simulink model "sampleModel242"  (R2021b)
settings: Solver=VariableStepAuto  StartTime=0.0  StopTime=10.0  RelTol=1e-3
undefined symbols (not defined in the file or in its folder): DiscIntNeverNeededParam
libraries: simulink x20, slpidlib x4
settings Model: Creator=user  LastModifiedBy=user

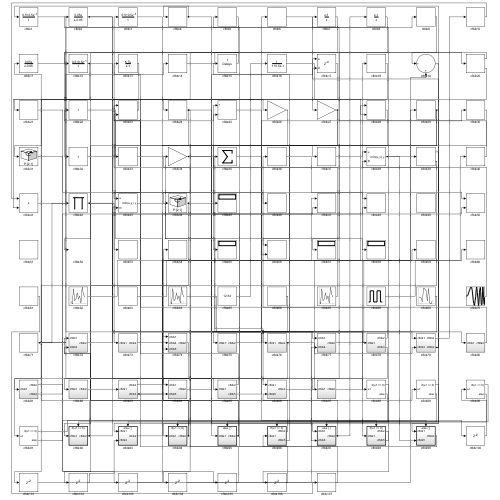
[thumbnail: Simulink's stored preview of the top-level diagram]
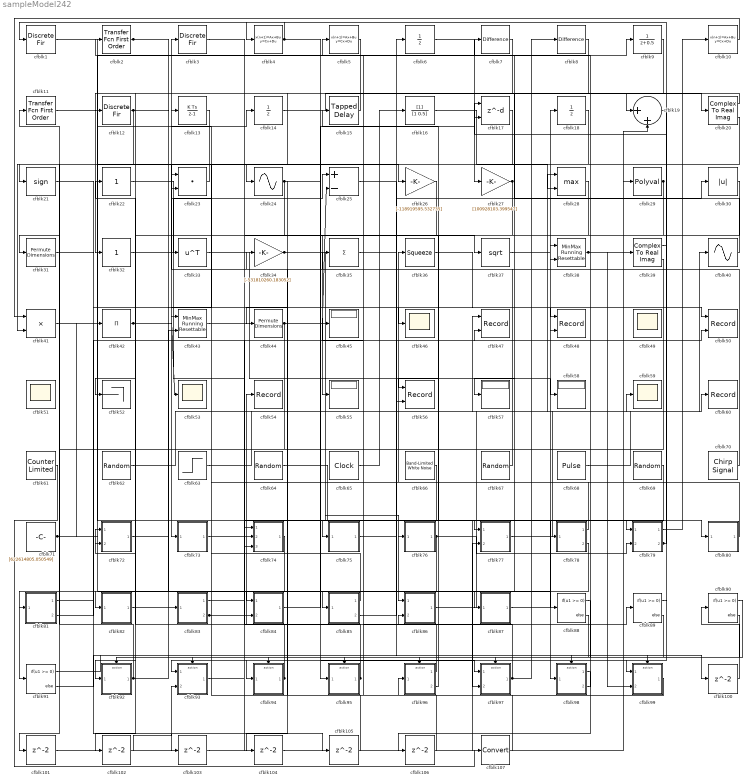
== system sampleModel242 ==
  cfblk1 : DiscreteFir  SampleTime=1
  cfblk10 : DiscreteStateSpace
  cfblk{100..106} (7 alike) : Delay  SampleTime=1
  cfblk107 : DataTypeConversion
  cfblk11 : simulink/Discrete/Transfer Fcn First Order  PoleZ=0.95  ICPrevOutput=0.0  DoSatur=off
  cfblk12 : DiscreteFir  SampleTime=1
  cfblk13 : DiscreteIntegrator  ICPrevOutput=DiscIntNeverNeededParam  ICPrevScaledInput=DiscIntNeverNeededParam
  cfblk14 : UnitDelay  HasFrameUpgradeWarning=on
  cfblk15 : simulink/Discrete/Tapped Delay  vinit=0.0  samptime=-1  NumDelays=1  DelayOrder=Oldest  includeCurrent=off
  cfblk16 : DiscreteFilter  SampleTime=1
  cfblk17 : Delay  DelayLengthSource=Input port  SampleTime=1
      settings: InputPortMap=u0,p1
  cfblk18 : UnitDelay  HasFrameUpgradeWarning=on
  cfblk19 : Sum  Inputs=|++
  cfblk2 : simulink/Discrete/Transfer Fcn First Order  PoleZ=0.95  ICPrevOutput=0.0  DoSatur=off
  cfblk20 : ComplexToRealImag
  cfblk21 : Signum
  cfblk22 : simulink/Math Operations/Slider Gain  gain=1  low=0  high=2
  cfblk23 : DotProduct  InputSameDT=on  OutDataTypeStr=Inherit: Inherit via internal rule
  cfblk24 : Sin  TimeSource=Use external signal  SampleTime=0
  cfblk25 : Sum  Inputs=+-
  cfblk26 : Gain  Gain=[-118919595.532735]
  cfblk27 : Gain  Gain=[100928103.399547]
  cfblk28 : MinMax  Function=max  Inputs=2
  cfblk29 : Polyval  Coefs=[ +2.081618890e-019, -1.441693666e-014, +4.719686976e-010, -8.536869453e-006, +1.621573104e-001, -8.087801117e+001 ]
  cfblk3 : DiscreteFir  SampleTime=1
  cfblk30 : Abs
  cfblk31 : PermuteDimensions
  cfblk32 : simulink/Math Operations/Slider Gain  gain=1  low=0  high=2
  cfblk33 : Math  Operator=transpose  SaturateOnIntegerOverflow=on
  cfblk34 : Gain  Gain=[-531810260.183052]
  cfblk35 : Sum  Inputs=+
  cfblk36 : Squeeze
  cfblk37 : Sqrt  SaturateOnIntegerOverflow=on
  cfblk38 : simulink/Math Operations/MinMax Running Resettable  Function=min  vinit=0.0
  cfblk39 : ComplexToRealImag
  cfblk4 : DiscreteStateSpace
  cfblk40 : Sin  TimeSource=Use external signal  SampleTime=0
  cfblk41 : Product  Inputs=**
  cfblk42 : Product  Inputs=*
  cfblk43 : simulink/Math Operations/MinMax Running Resettable  Function=min  vinit=0.0
  cfblk44 : PermuteDimensions
  cfblk{45,55,57..58} (4 alike) : Display
  cfblk{46,49,51,53,59} (5 alike) : Scope
      cfblk49 settings: Floating=on
      cfblk51 settings: Floating=on
  cfblk47 : Record  FileSettingsInternal="{\"entries\":[{\"content\":{\"excelSettings\":{\"content\":{},\"type\":\"Streamout.ExcelSettings\"}},\"type\":\"Streamout.FileSettingStorage\",\"uuid\":\"8466640d-3540-4ce9-993a-5f65f49446ff\"}],\"packageUris\":[\"http://schema.mathworks.com/mf0/streamout_blocks/R2020a\"],\"version\":\"1.0\"}"  Layout=[1 1]  SignalsInternal="{\"entries\":[{\"content\":{\"signals\":[{\"content\":{\"blockPath\":[\"sampleModel242/cfblk47\"],\"channel\":[],\"dimensions\":[1],\"domain\":\"sampleModel242/cfblk47\",\"lineColor\":\"#a2142f\",\"plots\":[1],\"port\":1,\"sid\":[\"\"],\"signalID\":9661,\"signalName\":\"cfblk63\"},\"type\":\"RecordBlkView.Signal\",\"uuid\":\"67ad4537-a0c7-4a78-aa5b-3ca15c563dde\"},{\"content\":{\"blockPath\":[\"sampleModel242/cfblk47\"],\"channel\":[],\"dimensions\":[1,1],\"domain\":\"sampleModel242/cfblk47\",\"lineColor\":\"#139fff\",\"plots\":[1],\"port\":2,\"sid\":[\"\"],\"signalID\":9665,\"signalName\":\"cfblk92\"},\"type\":\"RecordBlkView.Signal\",\"uuid\":\"e8972b09-f2da-4a53-9017-1d3f0a4a10ed\"}]},\"type\":\"RecordBlkView.InputSignals\",\"uuid\":\"aacada88-77af-4606-b280-0a5f38fbb807\"}],\"packageUris\":[\"http://schema.mathworks.com/mf0/streamout_blocks/R2020a\"],\"version\":\"1.0\"}"  VisualizationBindings="{\"xyplotplugin\":{\"info\":[{\"series\":[{\"bindingParametersList\":[{\"parameter\":\"X-Axis\",\"signalID\":9661,\"signalName\":\"cfblk63\"},{\"parameter\":\"Y-Axis\",\"signalID\":9665,\"signalName\":\"cfblk92\"}],\"seriesID\":40376}],\"subplotID\":1}]}}"  CompatibilityTag=XY
  cfblk48 : Record  FileSettingsInternal="{\"entries\":[{\"content\":{\"excelSettings\":{\"content\":{},\"type\":\"Streamout.ExcelSettings\"}},\"type\":\"Streamout.FileSettingStorage\",\"uuid\":\"c13b47bf-a8bf-41b9-80a1-0a6b1b0ceada\"}],\"packageUris\":[\"http://schema.mathworks.com/mf0/streamout_blocks/R2020a\"],\"version\":\"1.0\"}"  Layout=[1 1]  SignalsInternal="{\"entries\":[{\"content\":{\"signals\":[{\"content\":{\"blockPath\":[\"sampleModel242/cfblk48\"],\"channel\":[],\"dimensions\":[1,1],\"domain\":\"sampleModel242/cfblk48\",\"lineColor\":\"#a2142f\",\"plots\":[1],\"port\":1,\"sid\":[\"\"],\"signalID\":9669,\"signalName\":\"cfblk31\"},\"type\":\"RecordBlkView.Signal\",\"uuid\":\"329d8449-1276-47a0-bcc8-603c41fd3026\"},{\"content\":{\"blockPath\":[\"sampleModel242/cfblk48\"],\"channel\":[],\"dimensions\":[1],\"domain\":\"sampleModel242/cfblk48\",\"lineColor\":\"#139fff\",\"plots\":[1],\"port\":2,\"sid\":[\"\"],\"signalID\":9673,\"signalName\":\"cfblk83:2\"},\"type\":\"RecordBlkView.Signal\",\"uuid\":\"b307b965-bfc8-4c75-a60e-a0313d9c2b02\"}]},\"type\":\"RecordBlkView.InputSignals\",\"uuid\":\"3cab57f9-6900-416a-b86f-56591b424206\"}],\"packageUris\":[\"http://schema.mathworks.com/mf0/streamout_blocks/R2020a\"],\"version\":\"1.0\"}"  VisualizationBindings="{\"xyplotplugin\":{\"info\":[{\"series\":[{\"bindingParametersList\":[{\"parameter\":\"X-Axis\",\"signalID\":9669,\"signalName\":\"cfblk31\"},{\"parameter\":\"Y-Axis\",\"signalID\":9673,\"signalName\":\"cfblk83:2\"}],\"seriesID\":38915}],\"subplotID\":1}]}}"  CompatibilityTag=XY
  cfblk5 : DiscreteStateSpace
  cfblk50 : Record  FileSettingsInternal="{\"entries\":[{\"content\":{\"excelSettings\":{\"content\":{},\"type\":\"Streamout.ExcelSettings\"}},\"type\":\"Streamout.FileSettingStorage\",\"uuid\":\"6b25f1e0-3625-4cd8-9b2f-529eb5e0b0c7\"}],\"packageUris\":[\"http://schema.mathworks.com/mf0/streamout_blocks/R2020a\"],\"version\":\"1.0\"}"  Layout=[1 1]  SignalsInternal="{\"entries\":[{\"content\":{\"signals\":[{\"content\":{\"blockPath\":[\"sampleModel242/cfblk50\"],\"channel\":[],\"dimensions\":[1],\"domain\":\"sampleModel242/cfblk50\",\"lineColor\":\"#a2142f\",\"plots\":[1],\"port\":1,\"sid\":[\"\"],\"signalID\":9677,\"signalName\":\"cfblk36\"},\"type\":\"RecordBlkView.Signal\",\"uuid\":\"2faef9c5-9386-467e-8d00-879811eaf1a7\"},{\"content\":{\"blockPath\":[\"sampleModel242/cfblk50\"],\"channel\":[],\"dimensions\":[1],\"domain\":\"sampleModel242/cfblk50\",\"lineColor\":\"#139fff\",\"plots\":[1],\"port\":2,\"sid\":[\"\"],\"signalID\":9681,\"signalName\":\"cfblk81:2\"},\"type\":\"RecordBlkView.Signal\",\"uuid\":\"3fd7d5d3-1578-4a63-9d5f-ee0901e409a9\"}]},\"type\":\"RecordBlkView.InputSignals\",\"uuid\":\"3d327c85-3593-4bfd-8775-d910ec92d710\"}],\"packageUris\":[\"http://schema.mathworks.com/mf0/streamout_blocks/R2020a\"],\"version\":\"1.0\"}"  VisualizationBindings="{\"xyplotplugin\":{\"info\":[{\"series\":[{\"bindingParametersList\":[{\"parameter\":\"X-Axis\",\"signalID\":9677,\"signalName\":\"cfblk36\"},{\"parameter\":\"Y-Axis\",\"signalID\":9681,\"signalName\":\"cfblk81:2\"}],\"seriesID\":706}],\"subplotID\":1}]}}"  CompatibilityTag=XY
  cfblk52 : Terminator
  cfblk54 : Record  FileSettingsInternal="{\"entries\":[{\"content\":{\"excelSettings\":{\"content\":{},\"type\":\"Streamout.ExcelSettings\"}},\"type\":\"Streamout.FileSettingStorage\",\"uuid\":\"06190793-f5fc-415c-b838-8303df1b911b\"}],\"packageUris\":[\"http://schema.mathworks.com/mf0/streamout_blocks/R2020a\"],\"version\":\"1.0\"}"  SignalsInternal="{\"entries\":[{\"content\":{\"signals\":[{\"content\":{\"blockPath\":[\"sampleModel242/cfblk54\"],\"channel\":[],\"dimensions\":[1],\"domain\":\"sampleModel242/cfblk54\",\"lineColor\":\"#ff13a6\",\"plots\":[1],\"port\":1,\"sid\":[\"\"],\"signalID\":9685,\"signalName\":\"cfblk94\"},\"type\":\"RecordBlkView.Signal\",\"uuid\":\"6a6a1d66-a567-4c36-91e1-80c7a0c5bc7a\"}]},\"type\":\"RecordBlkView.InputSignals\",\"uuid\":\"c8db5507-b214-4169-ac9a-3b7f1f8d503c\"}],\"packageUris\":[\"http://schema.mathworks.com/mf0/streamout_blocks/R2020a\"],\"version\":\"1.0\"}"  VisualizationBindings="{\"sparklinesplugin\":{\"info\":[{\"bindingParametersList\":[],\"subplotID\":1}]}}"
  cfblk56 : Record  FileSettingsInternal="{\"entries\":[{\"content\":{\"excelSettings\":{\"content\":{},\"type\":\"Streamout.ExcelSettings\"}},\"type\":\"Streamout.FileSettingStorage\",\"uuid\":\"80c68350-c5d5-4745-a822-7bd470e9d639\"}],\"packageUris\":[\"http://schema.mathworks.com/mf0/streamout_blocks/R2020a\"],\"version\":\"1.0\"}"  Layout=[1 1]  SignalsInternal="{\"entries\":[{\"content\":{\"signals\":[{\"content\":{\"blockPath\":[\"sampleModel242/cfblk56\"],\"channel\":[],\"dimensions\":[1],\"domain\":\"sampleModel242/cfblk56\",\"lineColor\":\"#a2142f\",\"plots\":[1],\"port\":1,\"sid\":[\"\"],\"signalID\":9689,\"signalName\":\"cfblk29\"},\"type\":\"RecordBlkView.Signal\",\"uuid\":\"3f9a410f-4a9b-4b88-868e-e92ce524b347\"},{\"content\":{\"blockPath\":[\"sampleModel242/cfblk56\"],\"channel\":[],\"dimensions\":[1],\"domain\":\"sampleModel242/cfblk56\",\"lineColor\":\"#139fff\",\"plots\":[1],\"port\":2,\"sid\":[\"\"],\"signalID\":9693,\"signalName\":\"cfblk35\"},\"type\":\"RecordBlkView.Signal\",\"uuid\":\"47182436-db97-462b-940f-56f22781204b\"}]},\"type\":\"RecordBlkView.InputSignals\",\"uuid\":\"28bf4cd6-305f-4118-8603-ea67f9f3f1eb\"}],\"packageUris\":[\"http://schema.mathworks.com/mf0/streamout_blocks/R2020a\"],\"version\":\"1.0\"}"  VisualizationBindings="{\"xyplotplugin\":{\"info\":[{\"series\":[{\"bindingParametersList\":[{\"parameter\":\"X-Axis\",\"signalID\":9689,\"signalName\":\"cfblk29\"},{\"parameter\":\"Y-Axis\",\"signalID\":9693,\"signalName\":\"cfblk35\"}],\"seriesID\":40562}],\"subplotID\":1}]}}"  CompatibilityTag=XY
  cfblk6 : UnitDelay  HasFrameUpgradeWarning=on
  cfblk60 : Record  FileSettingsInternal="{\"entries\":[{\"content\":{\"excelSettings\":{\"content\":{},\"type\":\"Streamout.ExcelSettings\"}},\"type\":\"Streamout.FileSettingStorage\",\"uuid\":\"ac3e01c3-e921-4d05-880d-693c9b2be958\"}],\"packageUris\":[\"http://schema.mathworks.com/mf0/streamout_blocks/R2020a\"],\"version\":\"1.0\"}"  SignalsInternal="{\"entries\":[{\"content\":{\"signals\":[{\"content\":{\"blockPath\":[\"sampleModel242/cfblk60\"],\"channel\":[],\"dimensions\":[1],\"domain\":\"sampleModel242/cfblk60\",\"lineColor\":\"#77ac30\",\"plots\":[1],\"port\":1,\"sid\":[\"\"],\"signalID\":9657,\"signalName\":\"cfblk73\"},\"type\":\"RecordBlkView.Signal\",\"uuid\":\"ee10d19c-2b42-44d8-8030-24d641aff3a6\"}]},\"type\":\"RecordBlkView.InputSignals\",\"uuid\":\"6dbc1fc7-41f6-4a64-bb1e-672c8c773d34\"}],\"packageUris\":[\"http://schema.mathworks.com/mf0/streamout_blocks/R2020a\"],\"version\":\"1.0\"}"  VisualizationBindings="{\"sparklinesplugin\":{\"info\":[{\"bindingParametersList\":[],\"subplotID\":1}]}}"
  cfblk61 : simulink/Sources/Counter Limited  uplimit=[647.000000]  tsamp=-1
  cfblk62 : UniformRandomNumber  Minimum=[-3232928567.587387]  Maximum=[4444264149.465066]  Seed=[1192027.000000]  SampleTime=0.1
  cfblk63 : Step  Time=[34.000000]  Before=[160858895.694501]  After=[813002846.290973]  SampleTime=0
  cfblk64 : UniformRandomNumber  Minimum=[-4185575344.574016]  Maximum=[9583603799.572458]  Seed=[1929106.000000]  SampleTime=0.1
  cfblk65 : DigitalClock
  cfblk66 : simulink/Sources/Band-Limited White Noise  Cov=[5099447589.018917]  Ts=0.1  seed=[2237415079.000000]
  cfblk67 : UniformRandomNumber  Minimum=[-6418738320.620914]  Maximum=[7113492972.441939]  Seed=[24566985.000000]  SampleTime=0.1
  cfblk68 : DiscretePulseGenerator  PulseType=Time based  Amplitude=[-591785427.766708]  Period=[98460536.017098]  PulseWidth=5  PhaseDelay=[6.000000]
  cfblk69 : RandomNumber  Mean=[-20192.595669]  Variance=[90897.731430]  Seed=[204664879.000000]  SampleTime=0.1
  cfblk7 : simulink/Discrete/Difference  ICPrevInput=0.0  OutMin=[]  OutMax=[]  OutDataTypeStr=Inherit: Inherit via back propagation  OutDataType=fixdt(1, 16)  OutScaling=2^-10  DoSatur=off
  cfblk70 : simulink/Sources/Chirp Signal  f1=[289852911.748048]  T=[-202458346.103400]  f2=[153008503.739660]
  cfblk71 : Constant  Value=[622614805.050549]  SampleTime=1
  cfblk72 : Subsystem
  cfblk73 : Subsystem
  cfblk74 : Subsystem
  cfblk75 : Subsystem
  cfblk76 : Subsystem
  cfblk77 : Subsystem
  cfblk78 : Subsystem
  cfblk79 : Subsystem
  cfblk8 : simulink/Discrete/Difference  ICPrevInput=0.0  OutMin=[]  OutMax=[]  OutDataTypeStr=Inherit: Inherit via back propagation  OutDataType=fixdt(1, 16)  OutScaling=2^-10  DoSatur=off
  cfblk80 : Subsystem
  cfblk81 : Subsystem
  cfblk82 : Subsystem
  cfblk83 : Subsystem
  cfblk84 : Subsystem
  cfblk85 : Subsystem
  cfblk86 : Subsystem
  cfblk87 : Subsystem
  cfblk{88..91} (4 alike) : If  IfExpression=u1 >= 0  SampleTime=1
  cfblk9 : DiscreteTransferFcn  SampleTime=1
  cfblk92 : Subsystem  TreatAsAtomicUnit=on
  cfblk93 : Subsystem  TreatAsAtomicUnit=on
  cfblk94 : Subsystem  TreatAsAtomicUnit=on
  cfblk95 : Subsystem  TreatAsAtomicUnit=on
  cfblk96 : Subsystem  TreatAsAtomicUnit=on
  cfblk97 : Subsystem  TreatAsAtomicUnit=on
  cfblk98 : Subsystem  TreatAsAtomicUnit=on
  cfblk99 : Subsystem  TreatAsAtomicUnit=on
  wires:
  cfblk94/1(cfblk2) -> cfblk54/1, cfblk72/1(cfblk1)
  cfblk71/1 -> cfblk9/1, cfblk42/1, cfblk95/1(cfblk1)
  cfblk65/1 -> cfblk16/1
  cfblk79/1(cfblk2) -> cfblk10/1
  cfblk32/1 -> cfblk25/1
  cfblk41/1 -> cfblk14/1
  cfblk68/1 -> cfblk4/1
  cfblk23/1 -> cfblk21/1
  cfblk78/1(cfblk2) -> cfblk36/1
  cfblk3/1 -> cfblk37/1
  cfblk11/1 -> cfblk75/1(cfblk1)
  cfblk33/1 -> cfblk86/1(cfblk1)
  cfblk38/1 -> cfblk39/1, cfblk99/2(cfblk5)
  cfblk76/1(cfblk2) -> cfblk82/1(cfblk1), cfblk79/2(cfblk3)
  cfblk9/1 -> cfblk57/1
  cfblk5/1 -> cfblk32/1
  cfblk67/1 -> cfblk3/1
  cfblk13/1 -> cfblk31/1
  cfblk63/1 -> cfblk47/1
  cfblk74/1(cfblk2) -> cfblk84/1(cfblk1)
  cfblk29/1 -> cfblk56/1, cfblk76/1(cfblk1)
  cfblk1/1 -> cfblk26/1
  cfblk34/1 -> cfblk98/1(cfblk1), cfblk78/1(cfblk1)
  cfblk7/1 -> cfblk24/1
  cfblk8/1 -> cfblk52/1
  cfblk87/1(cfblk2) -> cfblk18/1
  cfblk39/1 -> cfblk93/1(cfblk1)
  cfblk62/1 -> cfblk29/1
  cfblk69/1 -> cfblk84/2(cfblk5)
  cfblk2/1 -> cfblk46/1, cfblk77/1(cfblk1)
  cfblk43/1 -> cfblk58/1
  cfblk75/1(cfblk2) -> cfblk6/1
  cfblk35/1 -> cfblk56/2
  cfblk26/1 -> cfblk73/1(cfblk1)
  cfblk6/1 -> cfblk27/1
  cfblk85/1(cfblk2) -> cfblk13/1
  cfblk42/1 -> cfblk53/1, cfblk79/1(cfblk1)
  cfblk36/1 -> cfblk50/1
  cfblk12/1 -> cfblk88/1, cfblk81/1(cfblk1)
  cfblk27/1 -> cfblk44/1, cfblk102/1
  cfblk86/1(cfblk2) -> cfblk28/1
  cfblk99/1(cfblk2) -> cfblk96/1(cfblk1)
  cfblk31/1 -> cfblk48/1
  cfblk96/1(cfblk2) -> cfblk86/2(cfblk5)
  cfblk82/1(cfblk2) -> cfblk83/1(cfblk1)
  cfblk83/1(cfblk2) -> cfblk85/1(cfblk1)
  cfblk20/1 -> cfblk19/1
  cfblk66/1 -> cfblk94/1(cfblk1)
  cfblk22/1 -> cfblk74/1(cfblk1)
  cfblk20/2 -> cfblk33/1
  cfblk15/1 -> cfblk12/1
  cfblk10/1 -> cfblk41/1
  cfblk4/1 -> cfblk1/1, cfblk80/1(cfblk1)
  cfblk83/2(cfblk3) -> cfblk89/1, cfblk48/2
  cfblk14/1 -> cfblk20/1
  cfblk28/1 -> cfblk55/1
  cfblk78/2(cfblk3) -> cfblk91/1
  cfblk39/2 -> cfblk92/1(cfblk1)
  cfblk80/1(cfblk2) -> cfblk23/1
  cfblk17/1 -> cfblk41/2
  cfblk37/1 -> cfblk38/1
  cfblk30/1 -> cfblk87/1(cfblk1)
  cfblk98/2(cfblk5) -> cfblk2/1
  cfblk85/2(cfblk5) -> cfblk30/1
  cfblk73/1(cfblk2) -> cfblk60/1
  cfblk16/1 -> cfblk28/2
  cfblk44/1 -> cfblk25/2, cfblk101/1
  cfblk84/1(cfblk2) -> cfblk17/1
  cfblk19/1 -> cfblk99/1(cfblk1)
  cfblk79/2(cfblk4) -> cfblk35/1, cfblk17/2
  cfblk96/2(cfblk5) -> cfblk15/1
  cfblk18/1 -> cfblk43/1
  cfblk72/1(cfblk2) -> cfblk43/2
  cfblk70/1 -> cfblk38/2
  cfblk95/1(cfblk2) -> cfblk22/1, cfblk72/2(cfblk3)
  cfblk40/1 -> cfblk7/1
  cfblk81/2(cfblk4) -> cfblk50/2
  cfblk97/1(cfblk2) -> cfblk45/1, cfblk8/1
  cfblk24/1 -> cfblk97/1(cfblk1), cfblk74/3(cfblk5), cfblk104/1
  cfblk77/1(cfblk2) -> cfblk40/1
  cfblk92/1(cfblk2) -> cfblk47/2, cfblk11/1
  cfblk93/1(cfblk2) -> cfblk59/1
  cfblk64/1 -> cfblk97/2(cfblk3)
  cfblk88/1 -> cfblk92/Action
  cfblk88/2 -> cfblk93/Action
  cfblk89/1 -> cfblk94/Action
  cfblk89/2 -> cfblk95/Action
  cfblk90/1 -> cfblk96/Action
  cfblk90/2 -> cfblk97/Action
  cfblk91/1 -> cfblk98/Action
  cfblk91/2 -> cfblk99/Action
  cfblk25/1 -> cfblk100/1
  cfblk100/1 -> cfblk90/1
  cfblk101/1 -> cfblk74/2(cfblk4)
  cfblk102/1 -> cfblk93/2(cfblk4)
  cfblk81/1(cfblk2) -> cfblk103/1
  cfblk103/1 -> cfblk19/2
  cfblk104/1 -> cfblk77/2(cfblk4)
  cfblk21/1 -> cfblk105/1
  cfblk105/1 -> cfblk23/2
  cfblk98/1(cfblk2) -> cfblk106/1
  cfblk106/1 -> cfblk34/1
  cfblk61/1 -> cfblk107/1
  cfblk107/1 -> cfblk5/1

== system sampleModel242/cfblk72 ==
  cfblk1 : Inport
  cfblk3 : Inport  Port=2
  cfblk2 : Outport
  wires:
  cfblk1/1 -> cfblk2/1

== system sampleModel242/cfblk73 ==
  cfblk1 : Inport
  cfblk3 : DiscreteFir  SampleTime=1
  cfblk4 : Sum  Inputs=+
  cfblk2 : Outport
  wires:
  cfblk4/1 -> cfblk3/1
  cfblk1/1 -> cfblk4/1
  cfblk3/1 -> cfblk2/1

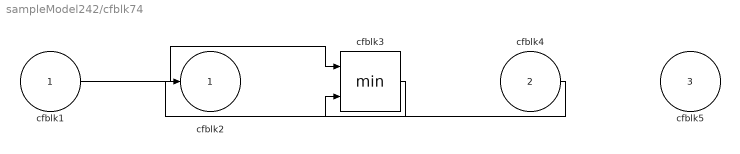
== system sampleModel242/cfblk74 ==
  cfblk1 : Inport
  cfblk4 : Inport  Port=2
  cfblk5 : Inport  Port=3
  cfblk3 : MinMax  Inputs=2
  cfblk2 : Outport
  wires:
  cfblk1/1 -> cfblk3/1
  cfblk3/1 -> cfblk2/1
  cfblk4/1 -> cfblk3/2

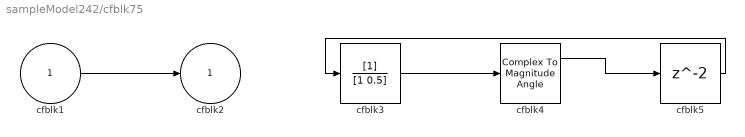
== system sampleModel242/cfblk75 ==
  cfblk1 : Inport
  cfblk3 : DiscreteFilter  SampleTime=1
  cfblk4 : ComplexToMagnitudeAngle
  cfblk5 : Delay  SampleTime=1
  cfblk2 : Outport
  wires:
  cfblk1/1 -> cfblk2/1
  cfblk3/1 -> cfblk4/1
  cfblk4/1 -> cfblk5/1
  cfblk5/1 -> cfblk3/1

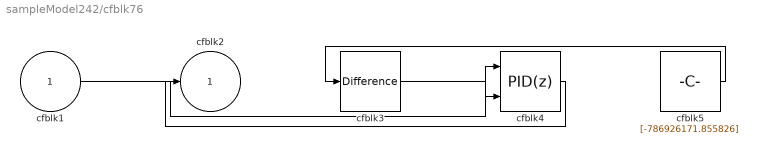
== system sampleModel242/cfblk76 ==
  cfblk1 : Inport
  cfblk3 : simulink/Discrete/Difference  ICPrevInput=0.0  OutMin=[]  OutMax=[]  OutDataTypeStr=Inherit: Inherit via back propagation  OutDataType=fixdt(1, 16)  OutScaling=2^-10  DoSatur=off
  cfblk4 : slpidlib/PID Controller (2DOF)  Controller=PID  Form=Parallel  TimeDomain=Discrete-time  UseExternalTs=off  SampleTime=1  IntegratorMethod=Forward Euler  FilterMethod=Forward Euler  ControllerParametersSource=internal  P=1  I=1  D=0  UseFilter=on  N=100  b=1  c=1  TunerSelectOption=Transfer Function Based (PID Tuner App)  InitialConditionSource=internal  InitialConditionForIntegrator=0  InitialConditionForFilter=0  DifferentiatorICPrevScaledInput=0  ExternalReset=none  TrackingMode=off  Kt=1  LimitOutput=off  SatLimitsSource=internal  UpperSaturationLimit=inf  LowerSaturationLimit=-inf  LinearizeAsGain=off  AntiWindupMode=none  Kb=1  POutMin=[]  POutMax=[]  IOutMin=[]  IOutMax=[]  DOutMin=[]  DOutMax=[]  NOutMin=[]  NOutMax=[]  bOutMin=[]  bOutMax=[]  cOutMin=[]  cOutMax=[]  SumOutMin=[]  SumOutMax=[]  SaturationOutMin=[]  SaturationOutMax=[]  PParamMin=[]  PParamMax=[]  IParamMin=[]  IParamMax=[]  DParamMin=[]  DParamMax=[]  NParamMin=[]  NParamMax=[]  bParamMin=[]  bParamMax=[]  cParamMin=[]  cParamMax=[]  KbParamMin=[]  KbParamMax=[]  KtParamMin=[]  KtParamMax=[]  KbOutMin=[]  KbOutMax=[]  KtOutMin=[]  KtOutMax=[]  IntegratorOutMin=[]  IntegratorOutMax=[]  FilterOutMin=[]  FilterOutMax=[]  SumI1OutMin=[]  SumI1OutMax=[]  SumI2OutMin=[]  SumI2OutMax=[]  SumI3OutMin=[]  SumI3OutMax=[]  SumI4OutMin=[]  SumI4OutMax=[]  SumDOutMin=[]  SumDOutMax=[]  Sum1OutMin=[]  Sum1OutMax=[]  Sum2OutMin=[]  Sum2OutMax=[]  Sum3OutMin=[]  Sum3OutMax=[]  DifferentiatorOutMin=[]  DifferentiatorOutMax=[]  FilterDiffOutCoefMin=[]  FilterDiffOutCoefMax=[]  ReciprocalOutMin=[]  ReciprocalOutMax=[]  SumDenOutMin=[]  SumDenOutMax=[]  SumNumOutMin=[]  SumNumOutMax=[]  DivideOutMin=[]  DivideOutMax=[]  UdiffTsProdOutMin=[]  UdiffTsProdOutMax=[]  NTsProdOutMin=[]  NTsProdOutMax=[]  UintegralTsProdOutMin=[]  UintegralTsProdOutMax=[]  UngainTsProdOutMin=[]  UngainTsProdOutMax=[]  IntegratorContinuousStateAttributes=''  IntegratorStateMustResolveToSignalObject=off  IntegratorRTWStateStorageClass=Auto  FilterContinuousStateAttributes=''  FilterStateMustResolveToSignalObject=off  FilterRTWStateStorageClass=Auto  ParallelPVariant=InternalParameters  IdealPVariant=Disabled  IVariant=InternalParameters  DVariant=InternalParameters  bVariant=InternalParameters  cVariant=InternalParameters  IntegratorVariant=Discrete  SatVariant=Disabled  AWVariant=Passthrough  PCopyVariant=Disabled  TRVariant=Disabled  FdbkBlocksVariant=Forward  IdealPFdbkVariant=Disabled  SatFdbkVariant=Disabled  DerivativeFilterVariant=ForwardEulerFilter  NVariant=InternalParameters  NCopyVariant=Disabled  FilterICVariant=InternalICsFilter  IntegratorICVariant=InternalICs  ExternalResetVariant=Disabled  TRSumVariant=Passthrough  SumFdbkVariant=Disabled  SumVariant=Sum_PID  TsampFilterVariant=InternalTs  TsampNgainVariant=Passthrough  TsampIntegralVariant=Passthrough  ExternalSaturationOutDataTypeStr=Inherit: Same as second input
      settings: SourceProductBaseCode=SL
  cfblk5 : Constant  Value=[-786926171.855826]  SampleTime=1
  cfblk2 : Outport
  wires:
  cfblk5/1 -> cfblk3/1
  cfblk1/1 -> cfblk4/1
  cfblk3/1 -> cfblk4/2
  cfblk4/1 -> cfblk2/1

== system sampleModel242/cfblk77 ==
  cfblk1 : Inport
  cfblk4 : Inport  Port=2
  cfblk3 : simulink/Math Operations/Slider Gain  gain=1  low=0  high=2
  cfblk2 : Outport
  wires:
  cfblk1/1 -> cfblk3/1
  cfblk4/1 -> cfblk2/1

== system sampleModel242/cfblk78 ==
  cfblk1 : Inport
  cfblk2 : Outport
  cfblk3 : Outport  Port=2
  wires:
  cfblk1/1 -> cfblk3/1, cfblk2/1

== system sampleModel242/cfblk79 ==
  cfblk1 : Inport
  cfblk3 : Inport  Port=2
  cfblk2 : Outport
  cfblk4 : Outport  Port=2
  wires:
  cfblk1/1 -> cfblk2/1
  cfblk3/1 -> cfblk4/1

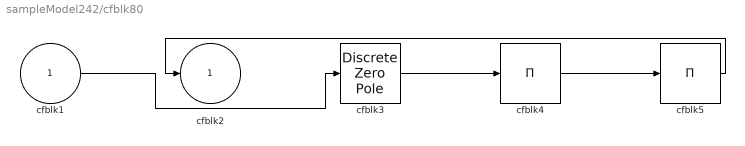
== system sampleModel242/cfblk80 ==
  cfblk1 : Inport
  cfblk3 : DiscreteZeroPole  Poles=[0 0.5]  Gain=1
  cfblk4 : Product  Inputs=*
  cfblk5 : Product  Inputs=*
  cfblk2 : Outport
  wires:
  cfblk5/1 -> cfblk2/1
  cfblk1/1 -> cfblk3/1
  cfblk3/1 -> cfblk4/1
  cfblk4/1 -> cfblk5/1

== system sampleModel242/cfblk81 ==
  cfblk1 : Inport
  cfblk3 : Delay  DelayLengthSource=Input port  SampleTime=1
      settings: InputPortMap=u0,p1
  cfblk2 : Outport
  cfblk4 : Outport  Port=2
  wires:
  cfblk1/1 -> cfblk3/1, cfblk2/1, cfblk3/2
  cfblk3/1 -> cfblk4/1

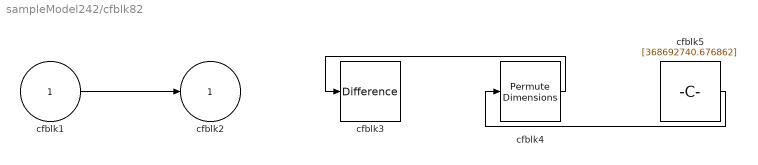
== system sampleModel242/cfblk82 ==
  cfblk1 : Inport
  cfblk3 : simulink/Discrete/Difference  ICPrevInput=0.0  OutMin=[]  OutMax=[]  OutDataTypeStr=Inherit: Inherit via back propagation  OutDataType=fixdt(1, 16)  OutScaling=2^-10  DoSatur=off
  cfblk4 : PermuteDimensions
  cfblk5 : Constant  Value=[368692740.676862]  SampleTime=1
  cfblk2 : Outport
  wires:
  cfblk1/1 -> cfblk2/1
  cfblk4/1 -> cfblk3/1
  cfblk5/1 -> cfblk4/1

== system sampleModel242/cfblk83 ==
  cfblk1 : Inport
  cfblk2 : Outport
  cfblk3 : Outport  Port=2
  wires:
  cfblk1/1 -> cfblk2/1, cfblk3/1

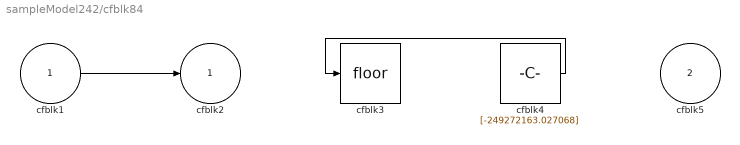
== system sampleModel242/cfblk84 ==
  cfblk1 : Inport
  cfblk5 : Inport  Port=2
  cfblk3 : Rounding
  cfblk4 : Constant  Value=[-249272163.027068]  SampleTime=1
  cfblk2 : Outport
  wires:
  cfblk1/1 -> cfblk2/1
  cfblk4/1 -> cfblk3/1

== system sampleModel242/cfblk85 ==
  cfblk1 : Inport
  cfblk3 : simulink/Discrete/Transfer Fcn Lead or Lag  PoleZ=0.95  ZeroZ=0.75  ICPrevOutput=0.0  ICPrevInput=0.0  DoSatur=off
      settings: SourceProductBaseCode=SL
  cfblk4 : Bias  Bias=[-871107666.530002]
  cfblk2 : Outport
  cfblk5 : Outport  Port=2
  wires:
  cfblk1/1 -> cfblk2/1, cfblk4/1
  cfblk4/1 -> cfblk3/1
  cfblk3/1 -> cfblk5/1

== system sampleModel242/cfblk86 ==
  cfblk1 : Inport
  cfblk5 : Inport  Port=2
  cfblk3 : slpidlib/PID Controller  Controller=PID  Form=Parallel  TimeDomain=Discrete-time  UseExternalTs=off  SampleTime=1  IntegratorMethod=Forward Euler  FilterMethod=Forward Euler  ControllerParametersSource=internal  P=1  I=1  D=0  UseFilter=on  N=100  TunerSelectOption=Transfer Function Based (PID Tuner App)  InitialConditionSource=internal  InitialConditionForIntegrator=0  InitialConditionForFilter=0  DifferentiatorICPrevScaledInput=0  ExternalReset=none  TrackingMode=off  Kt=1  LimitOutput=off  SatLimitsSource=internal  UpperSaturationLimit=inf  LowerSaturationLimit=-inf  LinearizeAsGain=off  AntiWindupMode=none  Kb=1  POutMin=[]  POutMax=[]  IOutMin=[]  IOutMax=[]  DOutMin=[]  DOutMax=[]  NOutMin=[]  NOutMax=[]  SumOutMin=[]  SumOutMax=[]  SaturationOutMin=[]  SaturationOutMax=[]  PParamMin=[]  PParamMax=[]  IParamMin=[]  IParamMax=[]  DParamMin=[]  DParamMax=[]  NParamMin=[]  NParamMax=[]  KbParamMin=[]  KbParamMax=[]  KtParamMin=[]  KtParamMax=[]  KbOutMin=[]  KbOutMax=[]  KtOutMin=[]  KtOutMax=[]  IntegratorOutMin=[]  IntegratorOutMax=[]  FilterOutMin=[]  FilterOutMax=[]  SumI1OutMin=[]  SumI1OutMax=[]  SumI2OutMin=[]  SumI2OutMax=[]  SumI3OutMin=[]  SumI3OutMax=[]  SumI4OutMin=[]  SumI4OutMax=[]  SumDOutMin=[]  SumDOutMax=[]  DifferentiatorOutMin=[]  DifferentiatorOutMax=[]  FilterDiffOutCoefMin=[]  FilterDiffOutCoefMax=[]  ReciprocalOutMin=[]  ReciprocalOutMax=[]  SumDenOutMin=[]  SumDenOutMax=[]  SumNumOutMin=[]  SumNumOutMax=[]  DivideOutMin=[]  DivideOutMax=[]  UdiffTsProdOutMin=[]  UdiffTsProdOutMax=[]  NTsProdOutMin=[]  NTsProdOutMax=[]  UintegralTsProdOutMin=[]  UintegralTsProdOutMax=[]  UngainTsProdOutMin=[]  UngainTsProdOutMax=[]  IntegratorContinuousStateAttributes=''  IntegratorStateMustResolveToSignalObject=off  IntegratorRTWStateStorageClass=Auto  FilterContinuousStateAttributes=''  FilterStateMustResolveToSignalObject=off  FilterRTWStateStorageClass=Auto  ParallelPVariant=InternalParameters  IdealPVariant=Disabled  IVariant=InternalParameters  DVariant=InternalParameters  IntegratorVariant=Discrete  SatVariant=Disabled  AWVariant=Passthrough  PCopyVariant=Disabled  TRVariant=Disabled  FdbkBlocksVariant=Forward  IdealPFdbkVariant=Disabled  SatFdbkVariant=Disabled  DerivativeFilterVariant=ForwardEulerFilter  NVariant=InternalParameters  NCopyVariant=Disabled  FilterICVariant=InternalICsFilter  IntegratorICVariant=InternalICs  ExternalResetVariant=Disabled  TRSumVariant=Passthrough  SumFdbkVariant=Disabled  SumVariant=Sum_PID  TsampFilterVariant=InternalTs  TsampNgainVariant=Passthrough  TsampIntegralVariant=Passthrough  ExternalSaturationOutDataTypeStr=Inherit: Same as second input
  cfblk4 : ComplexToMagnitudeAngle
  cfblk2 : Outport
  wires:
  cfblk1/1 -> cfblk2/1
  cfblk3/1 -> cfblk4/1
  cfblk5/1 -> cfblk3/1

== system sampleModel242/cfblk87 ==
  cfblk1 : Inport
  cfblk3 : PermuteDimensions
  cfblk4 : Sum  Inputs=+-
  cfblk5 : Constant  Value=[-851902695.866605]  SampleTime=1
  cfblk2 : Outport
  wires:
  cfblk5/1 -> cfblk4/1
  cfblk1/1 -> cfblk4/2
  cfblk3/1 -> cfblk2/1
  cfblk4/1 -> cfblk3/1

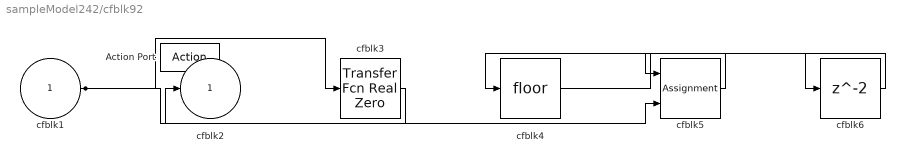
== system sampleModel242/cfblk92 ==
  cfblk1 : Inport
  Action Port : ActionPort  ActionPortLabel=if(u1 >= 0)
  cfblk3 : simulink/Discrete/Transfer Fcn Real Zero  ZeroZ=0.75  ICPrevInput=0.0  DoSatur=off
      settings: SourceProductBaseCode=SL
  cfblk4 : Rounding
  cfblk5 : Assignment  DiagnosticForDimensions=Warning  IndexOptions=Index vector (dialog)  Indices=1  OutputSizes=1
  cfblk6 : Delay
  cfblk2 : Outport
  wires:
  cfblk3/1 -> cfblk2/1
  cfblk1/1 -> cfblk3/1, cfblk5/2
  cfblk5/1 -> cfblk4/1
  cfblk4/1 -> cfblk6/1
  cfblk6/1 -> cfblk5/1

== system sampleModel242/cfblk93 ==
  cfblk1 : Inport
  cfblk4 : Inport  Port=2
  Action Port : ActionPort  ActionPortLabel=else
  cfblk3 : slpidlib/PID Controller  Controller=PID  Form=Parallel  TimeDomain=Discrete-time  UseExternalTs=off  SampleTime=-1  IntegratorMethod=Forward Euler  FilterMethod=Forward Euler  ControllerParametersSource=internal  P=1  I=1  D=0  UseFilter=on  N=100  TunerSelectOption=Transfer Function Based (PID Tuner App)  InitialConditionSource=internal  InitialConditionForIntegrator=0  InitialConditionForFilter=0  DifferentiatorICPrevScaledInput=0  ExternalReset=none  TrackingMode=off  Kt=1  LimitOutput=off  SatLimitsSource=internal  UpperSaturationLimit=inf  LowerSaturationLimit=-inf  LinearizeAsGain=off  AntiWindupMode=none  Kb=1  POutMin=[]  POutMax=[]  IOutMin=[]  IOutMax=[]  DOutMin=[]  DOutMax=[]  NOutMin=[]  NOutMax=[]  SumOutMin=[]  SumOutMax=[]  SaturationOutMin=[]  SaturationOutMax=[]  PParamMin=[]  PParamMax=[]  IParamMin=[]  IParamMax=[]  DParamMin=[]  DParamMax=[]  NParamMin=[]  NParamMax=[]  KbParamMin=[]  KbParamMax=[]  KtParamMin=[]  KtParamMax=[]  KbOutMin=[]  KbOutMax=[]  KtOutMin=[]  KtOutMax=[]  IntegratorOutMin=[]  IntegratorOutMax=[]  FilterOutMin=[]  FilterOutMax=[]  SumI1OutMin=[]  SumI1OutMax=[]  SumI2OutMin=[]  SumI2OutMax=[]  SumI3OutMin=[]  SumI3OutMax=[]  SumI4OutMin=[]  SumI4OutMax=[]  SumDOutMin=[]  SumDOutMax=[]  DifferentiatorOutMin=[]  DifferentiatorOutMax=[]  FilterDiffOutCoefMin=[]  FilterDiffOutCoefMax=[]  ReciprocalOutMin=[]  ReciprocalOutMax=[]  SumDenOutMin=[]  SumDenOutMax=[]  SumNumOutMin=[]  SumNumOutMax=[]  DivideOutMin=[]  DivideOutMax=[]  UdiffTsProdOutMin=[]  UdiffTsProdOutMax=[]  NTsProdOutMin=[]  NTsProdOutMax=[]  UintegralTsProdOutMin=[]  UintegralTsProdOutMax=[]  UngainTsProdOutMin=[]  UngainTsProdOutMax=[]  IntegratorContinuousStateAttributes=''  IntegratorStateMustResolveToSignalObject=off  IntegratorRTWStateStorageClass=Auto  FilterContinuousStateAttributes=''  FilterStateMustResolveToSignalObject=off  FilterRTWStateStorageClass=Auto  ParallelPVariant=InternalParameters  IdealPVariant=Disabled  IVariant=InternalParameters  DVariant=InternalParameters  IntegratorVariant=Discrete  SatVariant=Disabled  AWVariant=Passthrough  PCopyVariant=Disabled  TRVariant=Disabled  FdbkBlocksVariant=Forward  IdealPFdbkVariant=Disabled  SatFdbkVariant=Disabled  DerivativeFilterVariant=ForwardEulerFilter  NVariant=InternalParameters  NCopyVariant=Disabled  FilterICVariant=InternalICsFilter  IntegratorICVariant=InternalICs  ExternalResetVariant=Disabled  TRSumVariant=Passthrough  SumFdbkVariant=Disabled  SumVariant=Sum_PID  TsampFilterVariant=InternalTs  TsampNgainVariant=Passthrough  TsampIntegralVariant=Passthrough  ExternalSaturationOutDataTypeStr=Inherit: Same as second input
  cfblk2 : Outport
  wires:
  cfblk3/1 -> cfblk2/1
  cfblk4/1 -> cfblk3/1

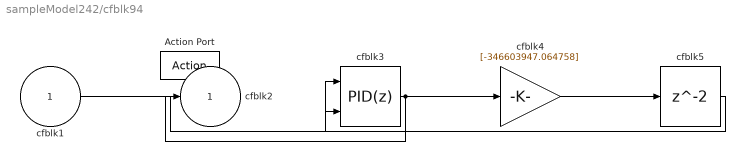
== system sampleModel242/cfblk94 ==
  cfblk1 : Inport
  Action Port : ActionPort  ActionPortLabel=if(u1 >= 0)
  cfblk3 : slpidlib/PID Controller (2DOF)  Controller=PID  Form=Parallel  TimeDomain=Discrete-time  UseExternalTs=off  SampleTime=-1  IntegratorMethod=Forward Euler  FilterMethod=Forward Euler  ControllerParametersSource=internal  P=1  I=1  D=0  UseFilter=on  N=100  b=1  c=1  TunerSelectOption=Transfer Function Based (PID Tuner App)  InitialConditionSource=internal  InitialConditionForIntegrator=0  InitialConditionForFilter=0  DifferentiatorICPrevScaledInput=0  ExternalReset=none  TrackingMode=off  Kt=1  LimitOutput=off  SatLimitsSource=internal  UpperSaturationLimit=inf  LowerSaturationLimit=-inf  LinearizeAsGain=off  AntiWindupMode=none  Kb=1  POutMin=[]  POutMax=[]  IOutMin=[]  IOutMax=[]  DOutMin=[]  DOutMax=[]  NOutMin=[]  NOutMax=[]  bOutMin=[]  bOutMax=[]  cOutMin=[]  cOutMax=[]  SumOutMin=[]  SumOutMax=[]  SaturationOutMin=[]  SaturationOutMax=[]  PParamMin=[]  PParamMax=[]  IParamMin=[]  IParamMax=[]  DParamMin=[]  DParamMax=[]  NParamMin=[]  NParamMax=[]  bParamMin=[]  bParamMax=[]  cParamMin=[]  cParamMax=[]  KbParamMin=[]  KbParamMax=[]  KtParamMin=[]  KtParamMax=[]  KbOutMin=[]  KbOutMax=[]  KtOutMin=[]  KtOutMax=[]  IntegratorOutMin=[]  IntegratorOutMax=[]  FilterOutMin=[]  FilterOutMax=[]  SumI1OutMin=[]  SumI1OutMax=[]  SumI2OutMin=[]  SumI2OutMax=[]  SumI3OutMin=[]  SumI3OutMax=[]  SumI4OutMin=[]  SumI4OutMax=[]  SumDOutMin=[]  SumDOutMax=[]  Sum1OutMin=[]  Sum1OutMax=[]  Sum2OutMin=[]  Sum2OutMax=[]  Sum3OutMin=[]  Sum3OutMax=[]  DifferentiatorOutMin=[]  DifferentiatorOutMax=[]  FilterDiffOutCoefMin=[]  FilterDiffOutCoefMax=[]  ReciprocalOutMin=[]  ReciprocalOutMax=[]  SumDenOutMin=[]  SumDenOutMax=[]  SumNumOutMin=[]  SumNumOutMax=[]  DivideOutMin=[]  DivideOutMax=[]  UdiffTsProdOutMin=[]  UdiffTsProdOutMax=[]  NTsProdOutMin=[]  NTsProdOutMax=[]  UintegralTsProdOutMin=[]  UintegralTsProdOutMax=[]  UngainTsProdOutMin=[]  UngainTsProdOutMax=[]  IntegratorContinuousStateAttributes=''  IntegratorStateMustResolveToSignalObject=off  IntegratorRTWStateStorageClass=Auto  FilterContinuousStateAttributes=''  FilterStateMustResolveToSignalObject=off  FilterRTWStateStorageClass=Auto  ParallelPVariant=InternalParameters  IdealPVariant=Disabled  IVariant=InternalParameters  DVariant=InternalParameters  bVariant=InternalParameters  cVariant=InternalParameters  IntegratorVariant=Discrete  SatVariant=Disabled  AWVariant=Passthrough  PCopyVariant=Disabled  TRVariant=Disabled  FdbkBlocksVariant=Forward  IdealPFdbkVariant=Disabled  SatFdbkVariant=Disabled  DerivativeFilterVariant=ForwardEulerFilter  NVariant=InternalParameters  NCopyVariant=Disabled  FilterICVariant=InternalICsFilter  IntegratorICVariant=InternalICs  ExternalResetVariant=Disabled  TRSumVariant=Passthrough  SumFdbkVariant=Disabled  SumVariant=Sum_PID  TsampFilterVariant=InternalTs  TsampNgainVariant=Passthrough  TsampIntegralVariant=Passthrough  ExternalSaturationOutDataTypeStr=Inherit: Same as second input
      settings: SourceProductBaseCode=SL
  cfblk4 : Gain  Gain=[-346603947.064758]
  cfblk5 : Delay
  cfblk2 : Outport
  wires:
  cfblk1/1 -> cfblk3/1
  cfblk3/1 -> cfblk2/1, cfblk4/1
  cfblk4/1 -> cfblk5/1
  cfblk5/1 -> cfblk3/2

== system sampleModel242/cfblk95 ==
  cfblk1 : Inport
  Action Port : ActionPort  ActionPortLabel=else
  cfblk3 : Squeeze
  cfblk2 : Outport
  wires:
  cfblk1/1 -> cfblk2/1, cfblk3/1

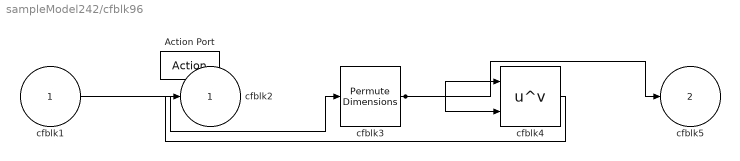
== system sampleModel242/cfblk96 ==
  cfblk1 : Inport
  Action Port : ActionPort  ActionPortLabel=if(u1 >= 0)
  cfblk3 : PermuteDimensions
  cfblk4 : Math  Operator=pow  SaturateOnIntegerOverflow=on
  cfblk2 : Outport
  cfblk5 : Outport  Port=2
  wires:
  cfblk3/1 -> cfblk5/1, cfblk4/1, cfblk4/2
  cfblk1/1 -> cfblk3/1
  cfblk4/1 -> cfblk2/1

== system sampleModel242/cfblk97 ==
  cfblk1 : Inport
  cfblk3 : Inport  Port=2
  Action Port : ActionPort  ActionPortLabel=else
  cfblk2 : Outport
  wires:
  cfblk1/1 -> cfblk2/1

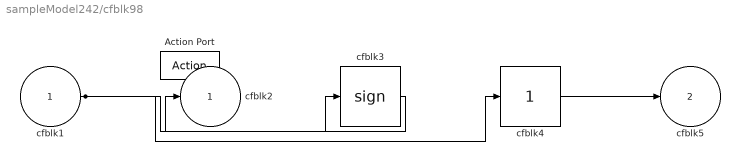
== system sampleModel242/cfblk98 ==
  cfblk1 : Inport
  Action Port : ActionPort  ActionPortLabel=if(u1 >= 0)
  cfblk3 : Signum
  cfblk4 : simulink/Math Operations/Slider Gain  gain=1  low=0  high=2
  cfblk2 : Outport
  cfblk5 : Outport  Port=2
  wires:
  cfblk3/1 -> cfblk2/1
  cfblk1/1 -> cfblk4/1, cfblk3/1
  cfblk4/1 -> cfblk5/1

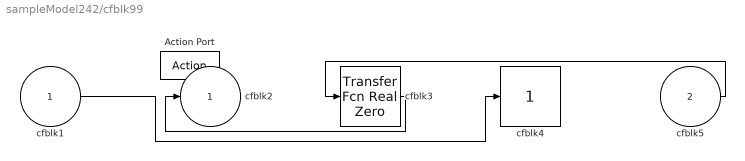
== system sampleModel242/cfblk99 ==
  cfblk1 : Inport
  cfblk5 : Inport  Port=2
  Action Port : ActionPort  ActionPortLabel=else
  cfblk3 : simulink/Discrete/Transfer Fcn Real Zero  ZeroZ=0.75  ICPrevInput=0.0  DoSatur=off
      settings: SourceProductBaseCode=SL
  cfblk4 : simulink/Math Operations/Slider Gain  gain=1  low=0  high=2
  cfblk2 : Outport
  wires:
  cfblk3/1 -> cfblk2/1
  cfblk5/1 -> cfblk3/1
  cfblk1/1 -> cfblk4/1
